simulink model "gm_lab2_floatp"  (R2022a)
settings: Solver=VariableStepAuto  StartTime=0.0  StopTime=10.0  RelTol=1e-3
settings Model: Creator=user  LastModifiedBy=user
settings OptimizationCC: BlockReduction=off  ConditionallyExecuteInputs=off
settings DebuggingCC: InheritedTsInSrcMsg=none

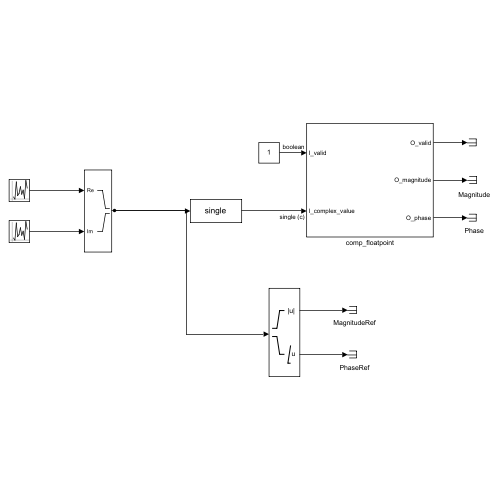
[thumbnail: Simulink's stored preview of the top-level diagram]
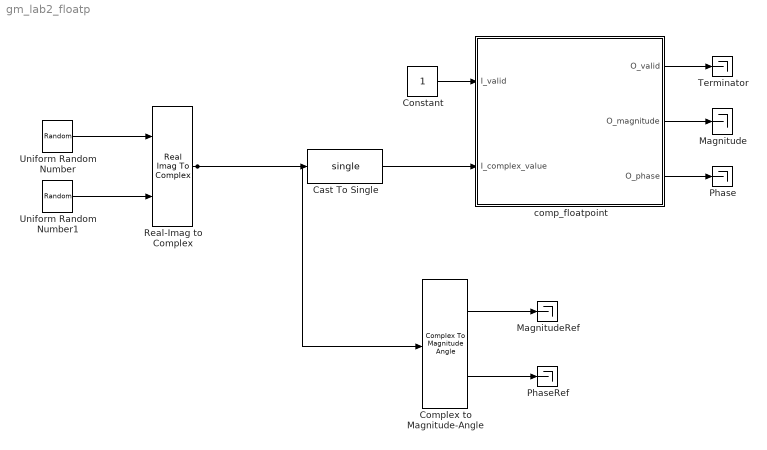
== system gm_lab2_floatp ==
  Cast To Single : DataTypeConversion  OutDataTypeStr=single  SaturateOnIntegerOverflow=off  RndMeth=Floor
  Complex to Magnitude-Angle : ComplexToMagnitudeAngle
  Constant : Constant  OutDataTypeStr=boolean  SampleTime=1
  Magnitude : Terminator
  MagnitudeRef : Terminator
  Phase : Terminator
  PhaseRef : Terminator
  Real-Imag to Complex : RealImagToComplex
  Terminator : Terminator
  Uniform Random Number : UniformRandomNumber  Minimum=0  Maximum=1023.99999976158142089844  Seed=10  SampleTime=1
  Uniform Random Number1 : UniformRandomNumber  Minimum=0  Maximum=1023.999999761581420898441  Seed=11  SampleTime=1
  comp_floatpoint : Subsystem
  wires:
  Complex to Magnitude-Angle/2 -> PhaseRef/1
  Complex to Magnitude-Angle/1 -> MagnitudeRef/1
  comp_floatpoint/2(O_magnitude) -> Magnitude/1
  comp_floatpoint/3(O_phase) -> Phase/1
  Cast To Single/1 -> comp_floatpoint/2(I_complex_value)
  comp_floatpoint/1(O_valid) -> Terminator/1
  Constant/1 -> comp_floatpoint/1(I_valid)
  Real-Imag to Complex/1 -> Complex to Magnitude-Angle/1, Cast To Single/1
  Uniform Random Number/1 -> Real-Imag to Complex/1
  Uniform Random Number1/1 -> Real-Imag to Complex/2

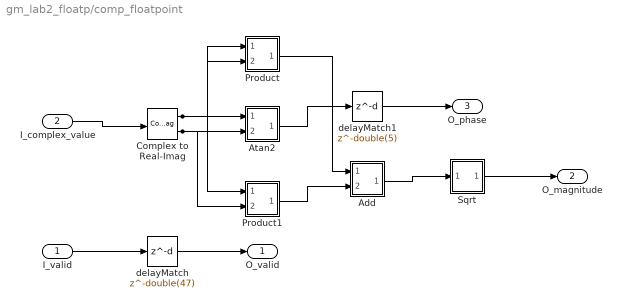
== system gm_lab2_floatp/comp_floatpoint ==
  I_valid : Inport  OutDataTypeStr=boolean  PortDimensions=1  SampleTime=1
  I_complex_value : Inport  Port=2  OutDataTypeStr=single  PortDimensions=1  SampleTime=1
      settings: SignalType=complex
  Add : Subsystem
      mask Display: disp('NFP\nadd');
  Atan2 : Subsystem
      mask Display: disp('NFP\ntrig3');
  Complex to Real-Imag : ComplexToRealImag  SampleTime=1
  Product : Subsystem
      mask Display: disp('NFP\nmul');
  Product1 : Subsystem
      mask Display: disp('NFP\nmul');
  Sqrt : Subsystem
      mask Display: disp('NFP\nsqrt');
  delayMatch : Delay  DelayLength=double(47)  InitialCondition=0  SampleTime=1
  delayMatch1 : Delay  DelayLength=double(5)  InitialCondition=0  SampleTime=1
  O_valid : Outport  SampleTime=1
  O_magnitude : Outport  Port=2  SampleTime=1
  O_phase : Outport  Port=3  SampleTime=1
  wires:
  delayMatch/1 -> O_valid/1
  I_complex_value/1 -> Complex to Real-Imag/1
  delayMatch1/1 -> O_phase/1
  Complex to Real-Imag/1 -> Product/2(In2), Product/1(In1), Atan2/2(In2)
  Complex to Real-Imag/2 -> Product1/2(In2), Product1/1(In1), Atan2/1(In1)
  Add/1(Out1) -> Sqrt/1(In1)
  Atan2/1(Out1) -> delayMatch1/1
  Product/1(Out1) -> Add/1(In1)
  Product1/1(Out1) -> Add/2(In2)
  Sqrt/1(Out1) -> O_magnitude/1
  I_valid/1 -> delayMatch/1

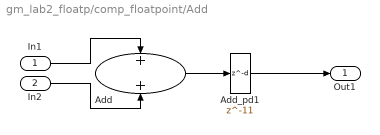
== system gm_lab2_floatp/comp_floatpoint/Add ==
  In1 : Inport
  In2 : Inport  Port=2
  Add : Sum  OutDataTypeStr=single  SampleTime=1
  Add_pd1 : Delay  DelayLength=11
  Out1 : Outport
  wires:
  In1/1 -> Add/1
  In2/1 -> Add/2
  Add/1 -> Add_pd1/1
  Add_pd1/1 -> Out1/1

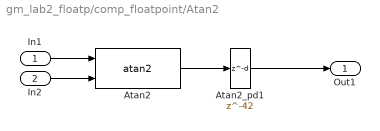
== system gm_lab2_floatp/comp_floatpoint/Atan2 ==
  In1 : Inport
  In2 : Inport  Port=2
  Atan2 : Trigonometry  Operator=atan2  SampleTime=1
  Atan2_pd1 : Delay  DelayLength=42
  Out1 : Outport
  wires:
  In1/1 -> Atan2/1
  In2/1 -> Atan2/2
  Atan2/1 -> Atan2_pd1/1
  Atan2_pd1/1 -> Out1/1

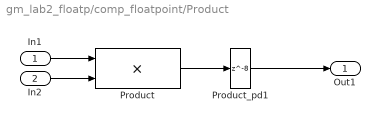
== system gm_lab2_floatp/comp_floatpoint/Product ==
  In1 : Inport
  In2 : Inport  Port=2
  Product : Product  Inputs=**  OutDataTypeStr=single  SampleTime=1
  Product_pd1 : Delay  DelayLength=8
  Out1 : Outport
  wires:
  In1/1 -> Product/1
  In2/1 -> Product/2
  Product/1 -> Product_pd1/1
  Product_pd1/1 -> Out1/1

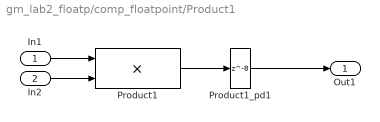
== system gm_lab2_floatp/comp_floatpoint/Product1 ==
  In1 : Inport
  In2 : Inport  Port=2
  Product1 : Product  Inputs=**  OutDataTypeStr=single  SampleTime=1
  Product1_pd1 : Delay  DelayLength=8
  Out1 : Outport
  wires:
  In1/1 -> Product1/1
  In2/1 -> Product1/2
  Product1/1 -> Product1_pd1/1
  Product1_pd1/1 -> Out1/1

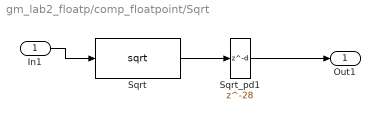
== system gm_lab2_floatp/comp_floatpoint/Sqrt ==
  In1 : Inport
  Sqrt : Sqrt  SampleTime=1
  Sqrt_pd1 : Delay  DelayLength=28
  Out1 : Outport
  wires:
  In1/1 -> Sqrt/1
  Sqrt/1 -> Sqrt_pd1/1
  Sqrt_pd1/1 -> Out1/1
